simulink model "QFTAxiLite"  (R2023b)
settings: Solver=VariableStepAuto  StartTime=0.0  StopTime=30  FixedStep=0.01  RelTol=1e-3
undefined symbols (not defined in the file): AXI4, i, Lite
libraries: hdlBasic x224, vmcUtilities x1
(part 1 of 2)
settings Model: Creator=finla  LastModifiedBy=finla

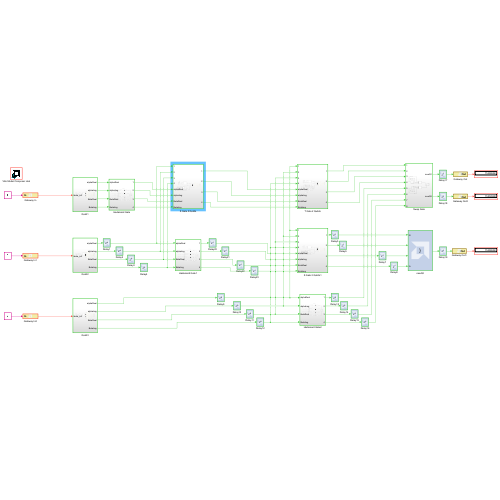
[thumbnail: Simulink's stored preview of the top-level diagram]
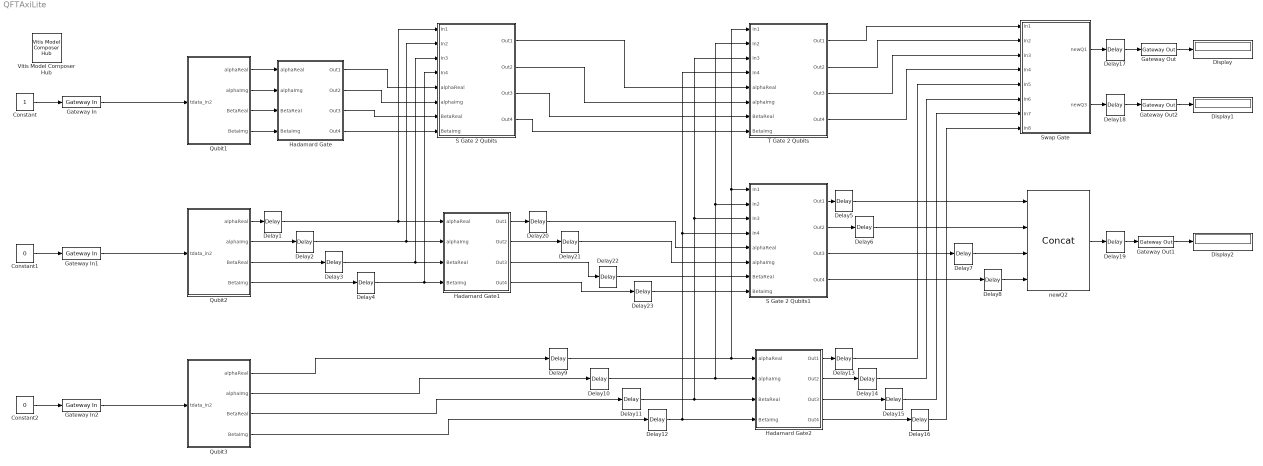
== system QFTAxiLite ==
  Constant : Constant
  Constant1 : Constant  Value=0
  Constant2 : Constant  Value=0
  Delay{1..4} (4 alike) : hdlBasic/Delay  rst=off  en=off  latency=4  reg_retiming=off  XmcBlockStatus=1  maskContainerNames=group1  block_type=delay  block_config=sysgen:Delay_config
  Delay{9..12} (4 alike) : hdlBasic/Delay  rst=off  en=off  latency=9  reg_retiming=off  XmcBlockStatus=1  maskContainerNames=group1  block_type=delay  block_config=sysgen:Delay_config
  Delay{13..16} (4 alike) : hdlBasic/Delay  rst=off  en=off  latency=2  reg_retiming=off  XmcBlockStatus=1  maskContainerNames=group1  block_type=delay  block_config=sysgen:Delay_config
  Delay{5..8,17..23} (11 alike) : hdlBasic/Delay  rst=off  en=off  latency=1  reg_retiming=off  XmcBlockStatus=1  maskContainerNames=group1  block_type=delay  block_config=sysgen:Delay_config
  Display : Display
  Display1 : Display
  Display2 : Display
  Gateway In : hdlBasic/Gateway In  gui_display_data_type=Fixed-point  arith_type=Unsigned  n_bits=32  bin_pt=0  preci_type=Single  exp_width=8  frac_width=24  rows=1  columns=1  quantization="Round  (unbiased: +/- Inf)"  overflow=Saturate  period=1  UseAsADC=off  ADCChannel='1'  interface=AXI4-Lite  automatic_assignment=on  address_offset=hex2dec('00')  intf_name=''  intf_description=''  default_value=0  timing_constraint=None  locs_specified=off  LOCs={}  io_standard={}  inherit_from_input=off  hdl_port=on  XmcBlockStatus=1  maskContainerNames=group4  block_type=gatewayin  block_config=sysgen:gateway_in_config  block_width_w=590  block_height_w=620  block_width=640  block_height=850
  Gateway In1 : hdlBasic/Gateway In  gui_display_data_type=Fixed-point  arith_type=Unsigned  n_bits=32  bin_pt=0  preci_type=Single  exp_width=8  frac_width=24  rows=1  columns=1  quantization="Round  (unbiased: +/- Inf)"  overflow=Saturate  period=1  UseAsADC=off  ADCChannel='1'  interface=AXI4-Lite  automatic_assignment=on  address_offset=hex2dec('00')  intf_name=''  intf_description=''  default_value=0  timing_constraint=None  locs_specified=off  LOCs={}  io_standard={}  inherit_from_input=off  hdl_port=on  XmcBlockStatus=1  maskContainerNames=group4  block_type=gatewayin  block_config=sysgen:gateway_in_config  block_width_w=590  block_height_w=620  block_width=640  block_height=850
  Gateway In2 : hdlBasic/Gateway In  gui_display_data_type=Fixed-point  arith_type=Unsigned  n_bits=32  bin_pt=0  preci_type=Single  exp_width=8  frac_width=24  rows=1  columns=1  quantization="Round  (unbiased: +/- Inf)"  overflow=Saturate  period=1  UseAsADC=off  ADCChannel='1'  interface=AXI4-Lite  automatic_assignment=on  address_offset=hex2dec('00')  intf_name=''  intf_description=''  default_value=0  timing_constraint=None  locs_specified=off  LOCs={}  io_standard={}  inherit_from_input=off  hdl_port=on  XmcBlockStatus=1  maskContainerNames=group4  block_type=gatewayin  block_config=sysgen:gateway_in_config  block_width_w=590  block_height_w=620  block_width=640  block_height=850
  Gateway Out : hdlBasic/Gateway Out  inherit_from_input=off  hdl_port=on  rows=1  columns=1  UseAsDAC=off  DACChannel='1'  interface=AXI4-Lite  automatic_assignment=on  address_offset=hex2dec('00')  intf_name=''  intf_description=''  timing_constraint=None  locs_specified=off  LOCs={}  io_standard={}  XmcBlockStatus=1  maskContainerNames=group4  block_type=gatewayout  block_config=sysgen:gateway_out_config  block_width_w=590  block_height_w=620  block_width=620  block_height=750
  Gateway Out1 : hdlBasic/Gateway Out  inherit_from_input=off  hdl_port=on  rows=1  columns=1  UseAsDAC=off  DACChannel='1'  interface=AXI4-Lite  automatic_assignment=on  address_offset=hex2dec('00')  intf_name=''  intf_description=''  timing_constraint=None  locs_specified=off  LOCs={}  io_standard={}  XmcBlockStatus=1  maskContainerNames=group4  block_type=gatewayout  block_config=sysgen:gateway_out_config  block_width_w=590  block_height_w=620  block_width=620  block_height=750
  Gateway Out2 : hdlBasic/Gateway Out  inherit_from_input=off  hdl_port=on  rows=1  columns=1  UseAsDAC=off  DACChannel='1'  interface=AXI4-Lite  automatic_assignment=on  address_offset=hex2dec('00')  intf_name=''  intf_description=''  timing_constraint=None  locs_specified=off  LOCs={}  io_standard={}  XmcBlockStatus=1  maskContainerNames=group4  block_type=gatewayout  block_config=sysgen:gateway_out_config  block_width_w=590  block_height_w=620  block_width=620  block_height=750
  Hadamard Gate : Subsystem
  Hadamard Gate1 : Subsystem
  Hadamard Gate2 : Subsystem
  Qubit1 : Subsystem
  Qubit2 : Subsystem
  Qubit3 : Subsystem
  S Gate 2 Qubits : Subsystem
  S Gate 2 Qubits1 : Subsystem
  Swap Gate : Subsystem
  T Gate 2 Qubits : Subsystem
  Vitis Model Composer Hub : vmcUtilities/Vitis Model Composer Hub  Tag=genX  CodeGeneration=off  SubsystemName=QFTAxiLite  CompilationType=HDLCompilation  ExportTypeV2=IP Catalog  TargetDirectory=C:/Users/finla/Documents/QuantumProject/GatesMCFiles/ThreeQubitQFT  exportDesign=off  analyzeDesign=on  validateDesignOnHw=off  ExportType=System Generator  IpVendor=xilinx.com  IpLibrary=hls  IpVersion=1.0  IpHWLanguage=Verilog  AieCompilerOptions={}  AieSimulatorOptions={}  CreateTestbench=off  TestbenchStackSize=10  RunRtlSim=off  RunCSim=off  RunAieSim=off  AieSimTimeout=50000  RunAieSimProfiling=off  LaunchVitisAnalyzer=off  PlotOutput=off  RunX86Sim=off  X86SimTimeout=10  GenHwImage=off  GenLibadfXo=off  GenHwValidationCode=off  PlatformType=Not Specified  HwSystemType=Baremetal  HwValidationTarget=hw  ProjDevice=xczu3eg-sbva484-1-i  ProjDevicePart=xczu3eg-sbva484-1-i  SamplePeriod=-1  ClockFrequency=200  DataPathParallelism=1  xilinxfamily=zynquplus  part=xczu3eg  speed=-1-i  package=sbva484  directory=C:/Users/finla/Documents/QuantumProject/GatesMCFiles/ThreeQubitQFT  testbench=on  incr_netlist=off  synthesis_tool=Vivado  clock_wrapper=Clock Enables  dbl_ovrd=According to Block Masks  dcm_input_clock_period=10  sysclk_period=10  simulink_period=1  eval_field=0  IPInfoJsonString="{\"HDLSubsystem\":{\"SubsystemName\":\"QFTAxiLite\",\"IPName\":\"axi_stream_template\",\"IPLibrary\":\"SysGen\",\"IPVendor\":\"strath.ac.uk\",\"IPVersion\":\"1.0\",\"TargetDirectory\":\"C:/Users/finla/Documents/QuantumProject/GatesMCFiles/ThreeQubitQFT\",\"SubsystemDir\":\"C:/Users/finla/Documents/QuantumProject/GatesMCFiles/ThreeQubitQFT\\\\ip\\\\QFTAxiLite\"},\"SubsystemTag\":\"HDLNode\"}"  LogFileName=''  NThreads=4
  newQ2 : hdlBasic/Concat  num_inputs=4  XmcBlockStatus=1  maskContainerNames=group1  block_type=concat  block_config=sysgen:Concat_config
  wires:
  Qubit2/1(alphaReal) -> Delay1/1
  Qubit3/3(BetaReal) -> Delay11/1
  Delay3/1 -> Hadamard Gate1/3(BetaReal), S Gate 2 Qubits/3(In3)
  Delay2/1 -> Hadamard Gate1/2(alphaImg), S Gate 2 Qubits/2(In2)
  T Gate 2 Qubits/3(Out3) -> Swap Gate/3(In3)
  Delay1/1 -> Hadamard Gate1/1(alphaReal), S Gate 2 Qubits/1(In1)
  Delay4/1 -> Hadamard Gate1/4(BetaImg), S Gate 2 Qubits/4(In4)
  newQ2/1 -> Delay19/1
  T Gate 2 Qubits/4(Out4) -> Swap Gate/4(In4)
  Hadamard Gate/1(Out1) -> S Gate 2 Qubits/5(alphaReal)
  Qubit1/1(alphaReal) -> Hadamard Gate/1(alphaReal)
  Qubit1/2(alphaImg) -> Hadamard Gate/2(alphaImg)
  Qubit3/4(BetaImg) -> Delay12/1
  S Gate 2 Qubits/1(Out1) -> T Gate 2 Qubits/5(alphaReal)
  Qubit1/3(BetaReal) -> Hadamard Gate/3(BetaReal)
  S Gate 2 Qubits/4(Out4) -> T Gate 2 Qubits/8(BetaImg)
  Swap Gate/2(newQ3) -> Delay18/1
  Qubit2/3(BetaReal) -> Delay3/1
  Gateway In1/1 -> Qubit2/1(tdata_in2)
  Hadamard Gate1/1(Out1) -> Delay20/1
  Qubit3/1(alphaReal) -> Delay9/1
  Hadamard Gate2/1(Out1) -> Delay13/1
  Gateway In/1 -> Qubit1/1(tdata_in2)
  Hadamard Gate2/3(Out3) -> Delay15/1
  Hadamard Gate2/2(Out2) -> Delay14/1
  Qubit1/4(BetaImg) -> Hadamard Gate/4(BetaImg)
  Delay10/1 -> Hadamard Gate2/2(alphaImg), S Gate 2 Qubits1/2(In2), T Gate 2 Qubits/2(In2)
  Hadamard Gate2/4(Out4) -> Delay16/1
  Qubit2/2(alphaImg) -> Delay2/1
  Hadamard Gate/3(Out3) -> S Gate 2 Qubits/7(BetaReal)
  Hadamard Gate/2(Out2) -> S Gate 2 Qubits/6(alphaImg)
  S Gate 2 Qubits/3(Out3) -> T Gate 2 Qubits/7(BetaReal)
  Delay11/1 -> Hadamard Gate2/3(BetaReal), S Gate 2 Qubits1/3(In3), T Gate 2 Qubits/3(In3)
  S Gate 2 Qubits/2(Out2) -> T Gate 2 Qubits/6(alphaImg)
  Delay12/1 -> Hadamard Gate2/4(BetaImg), S Gate 2 Qubits1/4(In4), T Gate 2 Qubits/4(In4)
  Hadamard Gate/4(Out4) -> S Gate 2 Qubits/8(BetaImg)
  Gateway In2/1 -> Qubit3/1(tdata_in2)
  Delay9/1 -> Hadamard Gate2/1(alphaReal), S Gate 2 Qubits1/1(In1), T Gate 2 Qubits/1(In1)
  Hadamard Gate1/2(Out2) -> Delay21/1
  Hadamard Gate1/4(Out4) -> Delay23/1
  Qubit3/2(alphaImg) -> Delay10/1
  Qubit2/4(BetaImg) -> Delay4/1
  Hadamard Gate1/3(Out3) -> Delay22/1
  Constant/1 -> Gateway In/1
  Constant1/1 -> Gateway In1/1
  Constant2/1 -> Gateway In2/1
  Gateway Out/1 -> Display/1
  Gateway Out2/1 -> Display1/1
  Gateway Out1/1 -> Display2/1
  Delay17/1 -> Gateway Out/1
  Delay18/1 -> Gateway Out2/1
  Delay19/1 -> Gateway Out1/1
  S Gate 2 Qubits1/1(Out1) -> Delay5/1
  S Gate 2 Qubits1/2(Out2) -> Delay6/1
  S Gate 2 Qubits1/3(Out3) -> Delay7/1
  S Gate 2 Qubits1/4(Out4) -> Delay8/1
  T Gate 2 Qubits/1(Out1) -> Swap Gate/1(In1)
  T Gate 2 Qubits/2(Out2) -> Swap Gate/2(In2)
  Delay13/1 -> Swap Gate/5(In5)
  Delay14/1 -> Swap Gate/6(In6)
  Delay15/1 -> Swap Gate/7(In7)
  Delay16/1 -> Swap Gate/8(In8)
  Swap Gate/1(newQ1) -> Delay17/1
  Delay20/1 -> S Gate 2 Qubits1/5(alphaReal)
  Delay21/1 -> S Gate 2 Qubits1/6(alphaImg)
  Delay22/1 -> S Gate 2 Qubits1/7(BetaReal)
  Delay23/1 -> S Gate 2 Qubits1/8(BetaImg)
  Delay5/1 -> newQ2/1
  Delay6/1 -> newQ2/2
  Delay7/1 -> newQ2/3
  Delay8/1 -> newQ2/4

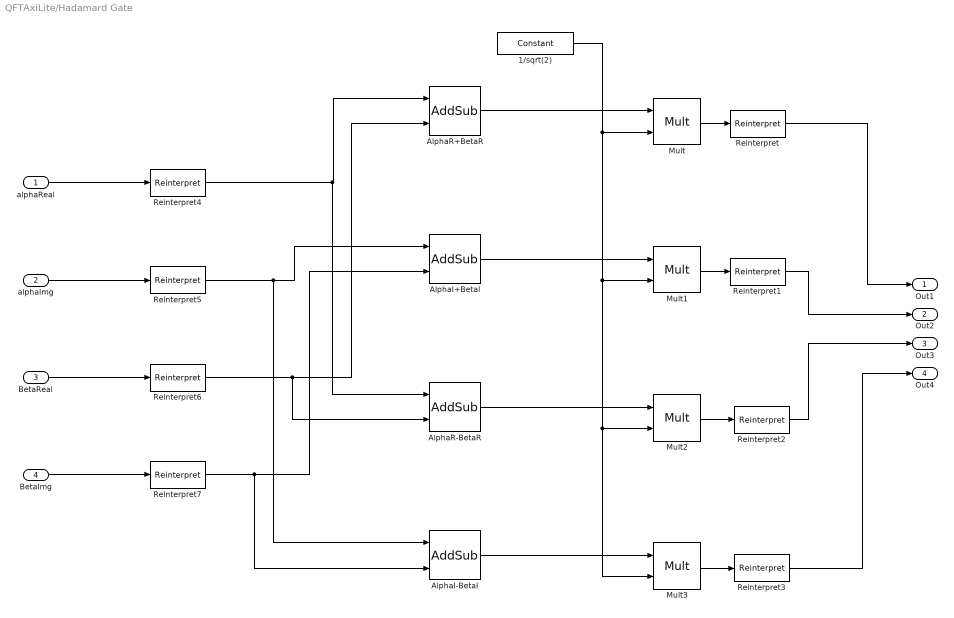
== system QFTAxiLite/Hadamard Gate ==
  alphaReal : Inport
  alphaImg : Inport  Port=2
  BetaReal : Inport  Port=3
  BetaImg : Inport  Port=4
  1/sqrt(2) : hdlBasic/Constant  const=1/sqrt(2)  gui_display_data_type=Fixed-point  arith_type=Signed (2's comp)  n_bits=16  bin_pt=13  preci_type=Single  exp_width=8  frac_width=24  explicit_period=on  period=1  XmcBlockStatus=1  maskContainerNames=tabcontainer1  block_type=constant  block_config=sysgen:Constant_config
  AlphaI+BetaI : hdlBasic/AddSub  mode=Addition  use_carryin=off  use_carryout=off  en=off  latency=1  precision=User Defined  arith_type="Signed  (2's comp)"  n_bits=8  bin_pt=0  quantization=Truncate  overflow=Saturate  use_behavioral_HDL=off  hw_selection=Fabric  pipelined=off  XmcBlockStatus=1  maskContainerNames=tabcontainer1  block_type=addsub  block_config=sysgen:Addsub_config
  AlphaI-BetaI : hdlBasic/AddSub  mode=Subtraction  use_carryin=off  use_carryout=off  en=off  latency=1  precision=User Defined  arith_type="Signed  (2's comp)"  n_bits=8  bin_pt=0  quantization=Truncate  overflow=Saturate  use_behavioral_HDL=off  hw_selection=Fabric  pipelined=off  XmcBlockStatus=1  maskContainerNames=tabcontainer1  block_type=addsub  block_config=sysgen:Addsub_config
  AlphaR+BetaR : hdlBasic/AddSub  mode=Addition  use_carryin=off  use_carryout=off  en=off  latency=1  precision=User Defined  arith_type="Signed  (2's comp)"  n_bits=8  bin_pt=0  quantization=Truncate  overflow=Saturate  use_behavioral_HDL=off  hw_selection=Fabric  pipelined=off  XmcBlockStatus=1  maskContainerNames=tabcontainer1  block_type=addsub  block_config=sysgen:Addsub_config
  AlphaR-BetaR : hdlBasic/AddSub  mode=Subtraction  use_carryin=off  use_carryout=off  en=off  latency=1  precision=User Defined  arith_type="Signed  (2's comp)"  n_bits=8  bin_pt=0  quantization=Truncate  overflow=Saturate  use_behavioral_HDL=off  hw_selection=Fabric  pipelined=off  XmcBlockStatus=1  maskContainerNames=tabcontainer1  block_type=addsub  block_config=sysgen:Addsub_config
  Mult{,1..3} (4 alike) : hdlBasic/Mult  precision=User Defined  arith_type="Signed  (2's comp)"  n_bits=8  bin_pt=6  quantization=Truncate  overflow=Flag as error  en=off  latency=3  use_behavioral_HDL=off  opt=Speed  use_embedded=on  optimum_pipeline=off  pipeline=on  use_rpm=on  placement_style=Triangular  XmcBlockStatus=1  maskContainerNames=group1  block_type=mult  block_config=sysgen:Mult_config  block_width=598  block_height=876
  Reinterpret{,1..3} (4 alike) : hdlBasic/Reinterpret  force_arith_type=on  arith_type=Unsigned  force_bin_pt=on  bin_pt=0  XmcBlockStatus=1  maskContainerNames=group1  block_type=reinterpret  block_config=sysgen:Reinterpret_config
  Reinterpret{4..7} (4 alike) : hdlBasic/Reinterpret  force_arith_type=on  arith_type="Signed  (2's comp)"  force_bin_pt=off  bin_pt=0  XmcBlockStatus=1  maskContainerNames=group1  block_type=reinterpret  block_config=sysgen:Reinterpret_config
  Out1 : Outport
  Out2 : Outport  Port=2
  Out3 : Outport  Port=3
  Out4 : Outport  Port=4
  wires:
  Reinterpret/1 -> Out1/1
  AlphaI-BetaI/1 -> Mult3/1
  Mult1/1 -> Reinterpret1/1
  Mult/1 -> Reinterpret/1
  Mult3/1 -> Reinterpret3/1
  Reinterpret3/1 -> Out4/1
  Reinterpret1/1 -> Out2/1
  AlphaR-BetaR/1 -> Mult2/1
  1/sqrt(2)/1 -> Mult3/2, Mult2/2, Mult1/2, Mult/2
  Reinterpret2/1 -> Out3/1
  AlphaI+BetaI/1 -> Mult1/1
  Mult2/1 -> Reinterpret2/1
  AlphaR+BetaR/1 -> Mult/1
  alphaReal/1 -> Reinterpret4/1
  alphaImg/1 -> Reinterpret5/1
  BetaReal/1 -> Reinterpret6/1
  BetaImg/1 -> Reinterpret7/1
  Reinterpret4/1 -> AlphaR-BetaR/1, AlphaR+BetaR/1
  Reinterpret5/1 -> AlphaI-BetaI/1, AlphaI+BetaI/1
  Reinterpret6/1 -> AlphaR-BetaR/2, AlphaR+BetaR/2
  Reinterpret7/1 -> AlphaI-BetaI/2, AlphaI+BetaI/2

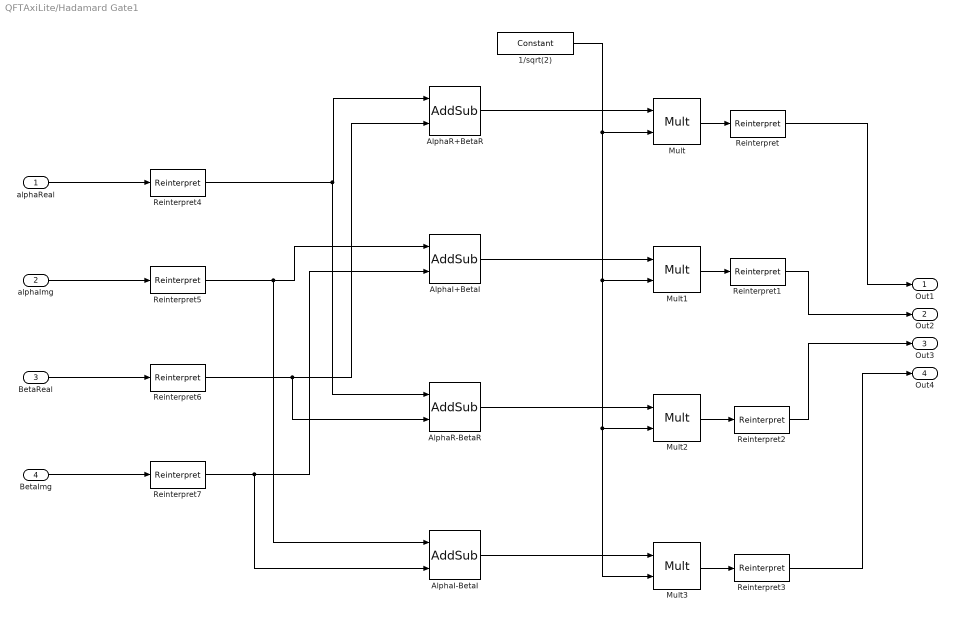
== system QFTAxiLite/Hadamard Gate1 ==
  alphaReal : Inport
  alphaImg : Inport  Port=2
  BetaReal : Inport  Port=3
  BetaImg : Inport  Port=4
  1/sqrt(2) : hdlBasic/Constant  const=1/sqrt(2)  gui_display_data_type=Fixed-point  arith_type=Signed (2's comp)  n_bits=16  bin_pt=13  preci_type=Single  exp_width=8  frac_width=24  explicit_period=on  period=1  XmcBlockStatus=1  maskContainerNames=tabcontainer1  block_type=constant  block_config=sysgen:Constant_config
  AlphaI+BetaI : hdlBasic/AddSub  mode=Addition  use_carryin=off  use_carryout=off  en=off  latency=1  precision=User Defined  arith_type="Signed  (2's comp)"  n_bits=8  bin_pt=0  quantization=Truncate  overflow=Saturate  use_behavioral_HDL=off  hw_selection=Fabric  pipelined=off  XmcBlockStatus=1  maskContainerNames=tabcontainer1  block_type=addsub  block_config=sysgen:Addsub_config
  AlphaI-BetaI : hdlBasic/AddSub  mode=Subtraction  use_carryin=off  use_carryout=off  en=off  latency=1  precision=User Defined  arith_type="Signed  (2's comp)"  n_bits=8  bin_pt=0  quantization=Truncate  overflow=Saturate  use_behavioral_HDL=off  hw_selection=Fabric  pipelined=off  XmcBlockStatus=1  maskContainerNames=tabcontainer1  block_type=addsub  block_config=sysgen:Addsub_config
  AlphaR+BetaR : hdlBasic/AddSub  mode=Addition  use_carryin=off  use_carryout=off  en=off  latency=1  precision=User Defined  arith_type="Signed  (2's comp)"  n_bits=8  bin_pt=0  quantization=Truncate  overflow=Saturate  use_behavioral_HDL=off  hw_selection=Fabric  pipelined=off  XmcBlockStatus=1  maskContainerNames=tabcontainer1  block_type=addsub  block_config=sysgen:Addsub_config
  AlphaR-BetaR : hdlBasic/AddSub  mode=Subtraction  use_carryin=off  use_carryout=off  en=off  latency=1  precision=User Defined  arith_type="Signed  (2's comp)"  n_bits=8  bin_pt=0  quantization=Truncate  overflow=Saturate  use_behavioral_HDL=off  hw_selection=Fabric  pipelined=off  XmcBlockStatus=1  maskContainerNames=tabcontainer1  block_type=addsub  block_config=sysgen:Addsub_config
  Mult{,1..3} (4 alike) : hdlBasic/Mult  precision=User Defined  arith_type="Signed  (2's comp)"  n_bits=8  bin_pt=6  quantization=Truncate  overflow=Flag as error  en=off  latency=3  use_behavioral_HDL=off  opt=Speed  use_embedded=on  optimum_pipeline=off  pipeline=on  use_rpm=on  placement_style=Triangular  XmcBlockStatus=1  maskContainerNames=group1  block_type=mult  block_config=sysgen:Mult_config  block_width=598  block_height=876
  Reinterpret{,1..3} (4 alike) : hdlBasic/Reinterpret  force_arith_type=on  arith_type=Unsigned  force_bin_pt=on  bin_pt=0  XmcBlockStatus=1  maskContainerNames=group1  block_type=reinterpret  block_config=sysgen:Reinterpret_config
  Reinterpret{4..7} (4 alike) : hdlBasic/Reinterpret  force_arith_type=on  arith_type="Signed  (2's comp)"  force_bin_pt=off  bin_pt=0  XmcBlockStatus=1  maskContainerNames=group1  block_type=reinterpret  block_config=sysgen:Reinterpret_config
  Out1 : Outport
  Out2 : Outport  Port=2
  Out3 : Outport  Port=3
  Out4 : Outport  Port=4
  wires:
  Reinterpret/1 -> Out1/1
  AlphaI-BetaI/1 -> Mult3/1
  Mult1/1 -> Reinterpret1/1
  Mult/1 -> Reinterpret/1
  Mult3/1 -> Reinterpret3/1
  Reinterpret3/1 -> Out4/1
  Reinterpret1/1 -> Out2/1
  AlphaR-BetaR/1 -> Mult2/1
  1/sqrt(2)/1 -> Mult3/2, Mult2/2, Mult1/2, Mult/2
  Reinterpret2/1 -> Out3/1
  AlphaI+BetaI/1 -> Mult1/1
  Mult2/1 -> Reinterpret2/1
  AlphaR+BetaR/1 -> Mult/1
  alphaReal/1 -> Reinterpret4/1
  alphaImg/1 -> Reinterpret5/1
  BetaReal/1 -> Reinterpret6/1
  BetaImg/1 -> Reinterpret7/1
  Reinterpret4/1 -> AlphaR-BetaR/1, AlphaR+BetaR/1
  Reinterpret5/1 -> AlphaI-BetaI/1, AlphaI+BetaI/1
  Reinterpret6/1 -> AlphaR-BetaR/2, AlphaR+BetaR/2
  Reinterpret7/1 -> AlphaI-BetaI/2, AlphaI+BetaI/2

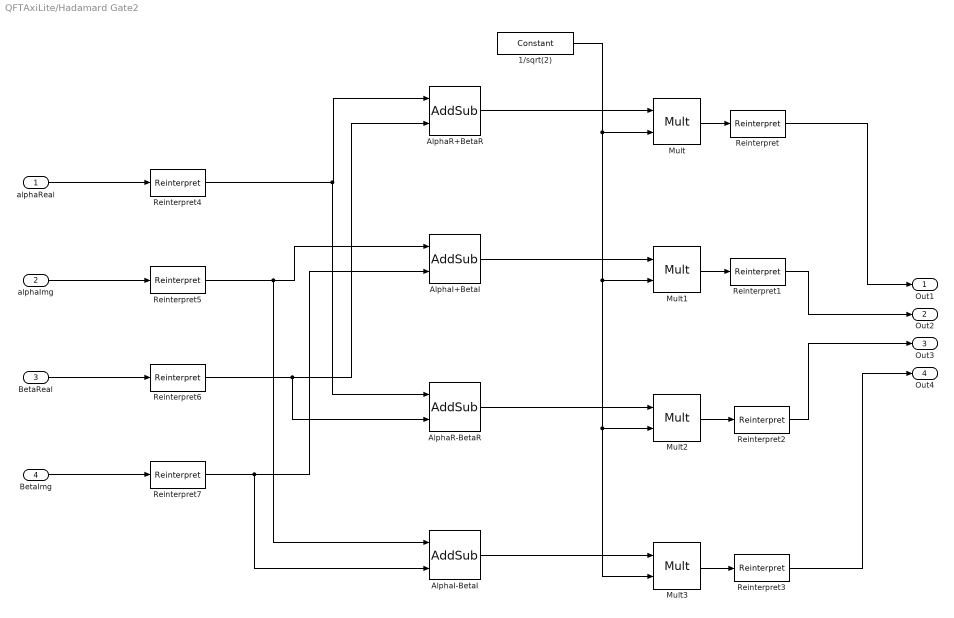
== system QFTAxiLite/Hadamard Gate2 ==
  alphaReal : Inport
  alphaImg : Inport  Port=2
  BetaReal : Inport  Port=3
  BetaImg : Inport  Port=4
  1/sqrt(2) : hdlBasic/Constant  const=1/sqrt(2)  gui_display_data_type=Fixed-point  arith_type=Signed (2's comp)  n_bits=16  bin_pt=13  preci_type=Single  exp_width=8  frac_width=24  explicit_period=on  period=1  XmcBlockStatus=1  maskContainerNames=tabcontainer1  block_type=constant  block_config=sysgen:Constant_config
  AlphaI+BetaI : hdlBasic/AddSub  mode=Addition  use_carryin=off  use_carryout=off  en=off  latency=1  precision=User Defined  arith_type="Signed  (2's comp)"  n_bits=8  bin_pt=0  quantization=Truncate  overflow=Saturate  use_behavioral_HDL=off  hw_selection=Fabric  pipelined=off  XmcBlockStatus=1  maskContainerNames=tabcontainer1  block_type=addsub  block_config=sysgen:Addsub_config
  AlphaI-BetaI : hdlBasic/AddSub  mode=Subtraction  use_carryin=off  use_carryout=off  en=off  latency=1  precision=User Defined  arith_type="Signed  (2's comp)"  n_bits=8  bin_pt=0  quantization=Truncate  overflow=Saturate  use_behavioral_HDL=off  hw_selection=Fabric  pipelined=off  XmcBlockStatus=1  maskContainerNames=tabcontainer1  block_type=addsub  block_config=sysgen:Addsub_config
  AlphaR+BetaR : hdlBasic/AddSub  mode=Addition  use_carryin=off  use_carryout=off  en=off  latency=1  precision=User Defined  arith_type="Signed  (2's comp)"  n_bits=8  bin_pt=0  quantization=Truncate  overflow=Saturate  use_behavioral_HDL=off  hw_selection=Fabric  pipelined=off  XmcBlockStatus=1  maskContainerNames=tabcontainer1  block_type=addsub  block_config=sysgen:Addsub_config
  AlphaR-BetaR : hdlBasic/AddSub  mode=Subtraction  use_carryin=off  use_carryout=off  en=off  latency=1  precision=User Defined  arith_type="Signed  (2's comp)"  n_bits=8  bin_pt=0  quantization=Truncate  overflow=Saturate  use_behavioral_HDL=off  hw_selection=Fabric  pipelined=off  XmcBlockStatus=1  maskContainerNames=tabcontainer1  block_type=addsub  block_config=sysgen:Addsub_config
  Mult{,1..3} (4 alike) : hdlBasic/Mult  precision=User Defined  arith_type="Signed  (2's comp)"  n_bits=8  bin_pt=6  quantization=Truncate  overflow=Flag as error  en=off  latency=3  use_behavioral_HDL=off  opt=Speed  use_embedded=on  optimum_pipeline=off  pipeline=on  use_rpm=on  placement_style=Triangular  XmcBlockStatus=1  maskContainerNames=group1  block_type=mult  block_config=sysgen:Mult_config  block_width=598  block_height=876
  Reinterpret{,1..3} (4 alike) : hdlBasic/Reinterpret  force_arith_type=on  arith_type=Unsigned  force_bin_pt=on  bin_pt=0  XmcBlockStatus=1  maskContainerNames=group1  block_type=reinterpret  block_config=sysgen:Reinterpret_config
  Reinterpret{4..7} (4 alike) : hdlBasic/Reinterpret  force_arith_type=on  arith_type="Signed  (2's comp)"  force_bin_pt=off  bin_pt=0  XmcBlockStatus=1  maskContainerNames=group1  block_type=reinterpret  block_config=sysgen:Reinterpret_config
  Out1 : Outport
  Out2 : Outport  Port=2
  Out3 : Outport  Port=3
  Out4 : Outport  Port=4
  wires:
  Reinterpret/1 -> Out1/1
  AlphaI-BetaI/1 -> Mult3/1
  Mult1/1 -> Reinterpret1/1
  Mult/1 -> Reinterpret/1
  Mult3/1 -> Reinterpret3/1
  Reinterpret3/1 -> Out4/1
  Reinterpret1/1 -> Out2/1
  AlphaR-BetaR/1 -> Mult2/1
  1/sqrt(2)/1 -> Mult3/2, Mult2/2, Mult1/2, Mult/2
  Reinterpret2/1 -> Out3/1
  AlphaI+BetaI/1 -> Mult1/1
  Mult2/1 -> Reinterpret2/1
  AlphaR+BetaR/1 -> Mult/1
  alphaReal/1 -> Reinterpret4/1
  alphaImg/1 -> Reinterpret5/1
  BetaReal/1 -> Reinterpret6/1
  BetaImg/1 -> Reinterpret7/1
  Reinterpret4/1 -> AlphaR-BetaR/1, AlphaR+BetaR/1
  Reinterpret5/1 -> AlphaI-BetaI/1, AlphaI+BetaI/1
  Reinterpret6/1 -> AlphaR-BetaR/2, AlphaR+BetaR/2
  Reinterpret7/1 -> AlphaI-BetaI/2, AlphaI+BetaI/2

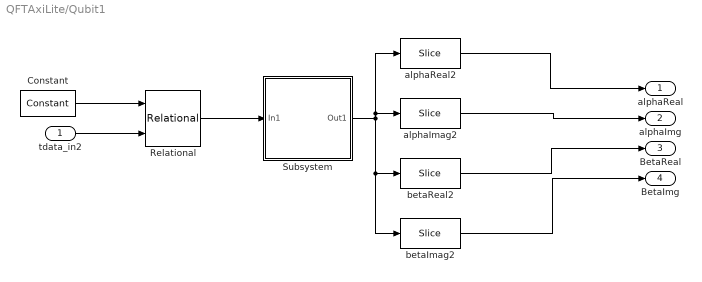
== system QFTAxiLite/Qubit1 ==
  tdata_in2 : Inport
  Constant : hdlBasic/Constant  const=0.0  gui_display_data_type=Fixed-point  arith_type=Unsigned  n_bits=32  bin_pt=0  preci_type=Single  exp_width=8  frac_width=24  explicit_period=off  period=1  XmcBlockStatus=1  maskContainerNames=tabcontainer1  block_type=constant  block_config=sysgen:Constant_config
  Relational : hdlBasic/Relational  mode=a=b  op_type=Unsigned Fix  en=off  latency=1  XmcBlockStatus=1  maskContainerNames=tabcontainer1  block_type=relational  block_config=sysgen:Relational_config
  Subsystem : Subsystem
  alphaImag2 : hdlBasic/Slice  nbits=16  boolean_output=off  mode=Two Bit Locations  bit1=23  base1=LSB of Input  bit0=16  base0=LSB of Input  XmcBlockStatus=1  maskContainerNames=group1  block_type=slice  block_config=sysgen:Slice_config
  alphaReal2 : hdlBasic/Slice  nbits=16  boolean_output=off  mode=Two Bit Locations  bit1=31  base1=LSB of Input  bit0=24  base0=LSB of Input  XmcBlockStatus=1  maskContainerNames=group1  block_type=slice  block_config=sysgen:Slice_config
  betaImag2 : hdlBasic/Slice  nbits=16  boolean_output=off  mode=Two Bit Locations  bit1=7  base1=LSB of Input  bit0=0  base0=LSB of Input  XmcBlockStatus=1  maskContainerNames=group1  block_type=slice  block_config=sysgen:Slice_config
  betaReal2 : hdlBasic/Slice  nbits=16  boolean_output=off  mode=Two Bit Locations  bit1=15  base1=LSB of Input  bit0=8  base0=LSB of Input  XmcBlockStatus=1  maskContainerNames=group1  block_type=slice  block_config=sysgen:Slice_config
  alphaReal : Outport
  alphaImg : Outport  Port=2
  BetaReal : Outport  Port=3
  BetaImg : Outport  Port=4
  wires:
  tdata_in2/1 -> Relational/2
  Constant/1 -> Relational/1
  Relational/1 -> Subsystem/1(In1)
  betaImag2/1 -> BetaImg/1
  betaReal2/1 -> BetaReal/1
  alphaReal2/1 -> alphaReal/1
  alphaImag2/1 -> alphaImg/1
  Subsystem/1(Out1) -> betaImag2/1, betaReal2/1, alphaImag2/1, alphaReal2/1

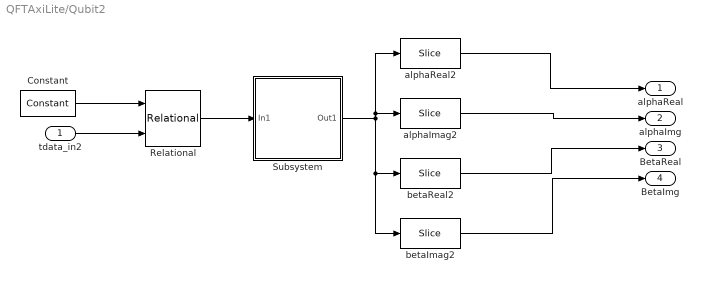
== system QFTAxiLite/Qubit2 ==
  tdata_in2 : Inport
  Constant : hdlBasic/Constant  const=0.0  gui_display_data_type=Fixed-point  arith_type=Unsigned  n_bits=32  bin_pt=0  preci_type=Single  exp_width=8  frac_width=24  explicit_period=off  period=1  XmcBlockStatus=1  maskContainerNames=tabcontainer1  block_type=constant  block_config=sysgen:Constant_config
  Relational : hdlBasic/Relational  mode=a=b  op_type=Unsigned Fix  en=off  latency=1  XmcBlockStatus=1  maskContainerNames=tabcontainer1  block_type=relational  block_config=sysgen:Relational_config
  Subsystem : Subsystem
  alphaImag2 : hdlBasic/Slice  nbits=16  boolean_output=off  mode=Two Bit Locations  bit1=23  base1=LSB of Input  bit0=16  base0=LSB of Input  XmcBlockStatus=1  maskContainerNames=group1  block_type=slice  block_config=sysgen:Slice_config
  alphaReal2 : hdlBasic/Slice  nbits=16  boolean_output=off  mode=Two Bit Locations  bit1=31  base1=LSB of Input  bit0=24  base0=LSB of Input  XmcBlockStatus=1  maskContainerNames=group1  block_type=slice  block_config=sysgen:Slice_config
  betaImag2 : hdlBasic/Slice  nbits=16  boolean_output=off  mode=Two Bit Locations  bit1=7  base1=LSB of Input  bit0=0  base0=LSB of Input  XmcBlockStatus=1  maskContainerNames=group1  block_type=slice  block_config=sysgen:Slice_config
  betaReal2 : hdlBasic/Slice  nbits=16  boolean_output=off  mode=Two Bit Locations  bit1=15  base1=LSB of Input  bit0=8  base0=LSB of Input  XmcBlockStatus=1  maskContainerNames=group1  block_type=slice  block_config=sysgen:Slice_config
  alphaReal : Outport
  alphaImg : Outport  Port=2
  BetaReal : Outport  Port=3
  BetaImg : Outport  Port=4
  wires:
  tdata_in2/1 -> Relational/2
  Constant/1 -> Relational/1
  Relational/1 -> Subsystem/1(In1)
  betaImag2/1 -> BetaImg/1
  betaReal2/1 -> BetaReal/1
  alphaReal2/1 -> alphaReal/1
  alphaImag2/1 -> alphaImg/1
  Subsystem/1(Out1) -> betaImag2/1, betaReal2/1, alphaImag2/1, alphaReal2/1

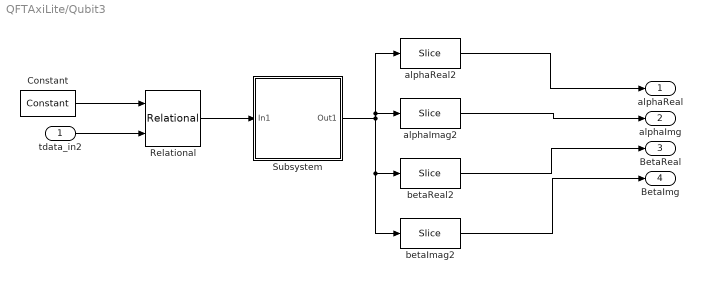
== system QFTAxiLite/Qubit3 ==
  tdata_in2 : Inport
  Constant : hdlBasic/Constant  const=0.0  gui_display_data_type=Fixed-point  arith_type=Unsigned  n_bits=32  bin_pt=0  preci_type=Single  exp_width=8  frac_width=24  explicit_period=off  period=1  XmcBlockStatus=1  maskContainerNames=tabcontainer1  block_type=constant  block_config=sysgen:Constant_config
  Relational : hdlBasic/Relational  mode=a=b  op_type=Unsigned Fix  en=off  latency=1  XmcBlockStatus=1  maskContainerNames=tabcontainer1  block_type=relational  block_config=sysgen:Relational_config
  Subsystem : Subsystem
  alphaImag2 : hdlBasic/Slice  nbits=16  boolean_output=off  mode=Two Bit Locations  bit1=23  base1=LSB of Input  bit0=16  base0=LSB of Input  XmcBlockStatus=1  maskContainerNames=group1  block_type=slice  block_config=sysgen:Slice_config
  alphaReal2 : hdlBasic/Slice  nbits=16  boolean_output=off  mode=Two Bit Locations  bit1=31  base1=LSB of Input  bit0=24  base0=LSB of Input  XmcBlockStatus=1  maskContainerNames=group1  block_type=slice  block_config=sysgen:Slice_config
  betaImag2 : hdlBasic/Slice  nbits=16  boolean_output=off  mode=Two Bit Locations  bit1=7  base1=LSB of Input  bit0=0  base0=LSB of Input  XmcBlockStatus=1  maskContainerNames=group1  block_type=slice  block_config=sysgen:Slice_config
  betaReal2 : hdlBasic/Slice  nbits=16  boolean_output=off  mode=Two Bit Locations  bit1=15  base1=LSB of Input  bit0=8  base0=LSB of Input  XmcBlockStatus=1  maskContainerNames=group1  block_type=slice  block_config=sysgen:Slice_config
  alphaReal : Outport
  alphaImg : Outport  Port=2
  BetaReal : Outport  Port=3
  BetaImg : Outport  Port=4
  wires:
  tdata_in2/1 -> Relational/2
  Constant/1 -> Relational/1
  Relational/1 -> Subsystem/1(In1)
  betaImag2/1 -> BetaImg/1
  betaReal2/1 -> BetaReal/1
  alphaReal2/1 -> alphaReal/1
  alphaImag2/1 -> alphaImg/1
  Subsystem/1(Out1) -> betaImag2/1, betaReal2/1, alphaImag2/1, alphaReal2/1

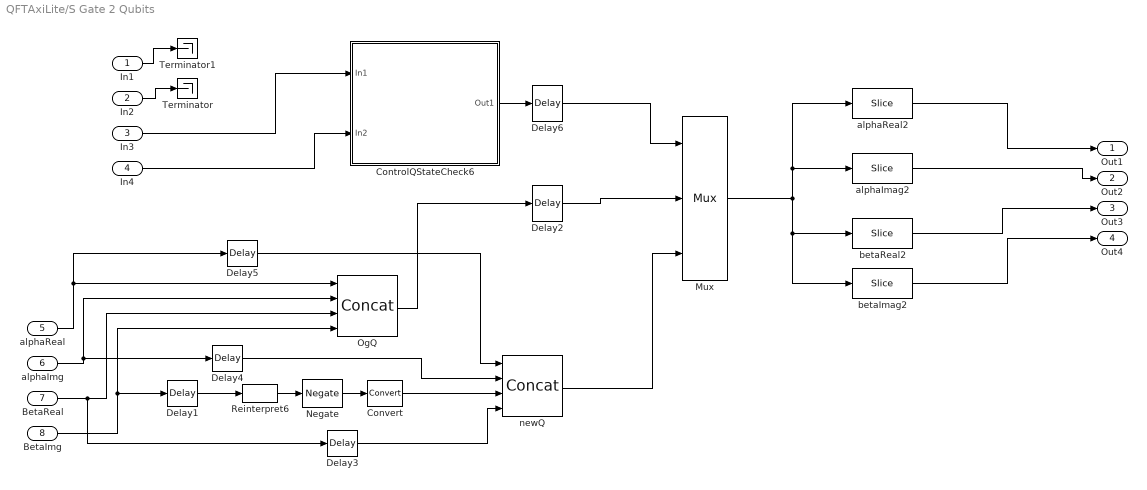
== system QFTAxiLite/S Gate 2 Qubits ==
  In1 : Inport
  In2 : Inport  Port=2
  In3 : Inport  Port=3
  In4 : Inport  Port=4
  alphaReal : Inport  Port=5
  alphaImg : Inport  Port=6
  BetaReal : Inport  Port=7
  BetaImg : Inport  Port=8
  ControlQStateCheck6 : Subsystem
  Convert : hdlBasic/Convert  gui_display_data_type=Fixed-point  arith_type=Unsigned  n_bits=8  bin_pt=0  float_type=Single  exp_bits=8  fraction_bits=24  quantization=Truncate  overflow=Wrap  en=off  latency=1  pipeline=off  XmcBlockStatus=1  maskContainerNames=group2  block_type=convert  block_config=sysgen:Convert_config  block_width=595  block_height=885
  Delay1 : hdlBasic/Delay  rst=off  en=off  latency=2  reg_retiming=off  XmcBlockStatus=1  maskContainerNames=group1  block_type=delay  block_config=sysgen:Delay_config
  Delay{2..5} (4 alike) : hdlBasic/Delay  rst=off  en=off  latency=4  reg_retiming=off  XmcBlockStatus=1  maskContainerNames=group1  block_type=delay  block_config=sysgen:Delay_config
  Delay6 : hdlBasic/Delay  rst=off  en=off  latency=1  reg_retiming=off  XmcBlockStatus=1  maskContainerNames=group1  block_type=delay  block_config=sysgen:Delay_config
  Mux : hdlBasic/Mux  inputs=2  en=off  latency=1  precision=Full  arith_type=Unsigned  n_bits=16  bin_pt=14  quantization=Truncate  overflow=Wrap  XmcBlockStatus=1  maskContainerNames=tabcontainer1  block_type=mux  block_config=sysgen:Mux_config
  Negate : hdlBasic/Negate  precision=Full  arith_type=Unsigned  n_bits=16  bin_pt=14  quantization=Truncate  overflow=Wrap  en=off  latency=1  XmcBlockStatus=1  maskContainerNames=tabcontainer1  block_type=negate  block_config=sysgen:Negate_config
  OgQ : hdlBasic/Concat  num_inputs=4  XmcBlockStatus=1  maskContainerNames=group1  block_type=concat  block_config=sysgen:Concat_config
  Reinterpret6 : hdlBasic/Reinterpret  force_arith_type=on  arith_type="Signed  (2's comp)"  force_bin_pt=off  bin_pt=0  XmcBlockStatus=1  maskContainerNames=group1  block_type=reinterpret  block_config=sysgen:Reinterpret_config
  Terminator : Terminator
  Terminator1 : Terminator
  alphaImag2 : hdlBasic/Slice  nbits=16  boolean_output=off  mode=Two Bit Locations  bit1=23  base1=LSB of Input  bit0=16  base0=LSB of Input  XmcBlockStatus=1  maskContainerNames=group1  block_type=slice  block_config=sysgen:Slice_config
  alphaReal2 : hdlBasic/Slice  nbits=16  boolean_output=off  mode=Two Bit Locations  bit1=31  base1=LSB of Input  bit0=24  base0=LSB of Input  XmcBlockStatus=1  maskContainerNames=group1  block_type=slice  block_config=sysgen:Slice_config
  betaImag2 : hdlBasic/Slice  nbits=16  boolean_output=off  mode=Two Bit Locations  bit1=7  base1=LSB of Input  bit0=0  base0=LSB of Input  XmcBlockStatus=1  maskContainerNames=group1  block_type=slice  block_config=sysgen:Slice_config
  betaReal2 : hdlBasic/Slice  nbits=16  boolean_output=off  mode=Two Bit Locations  bit1=15  base1=LSB of Input  bit0=8  base0=LSB of Input  XmcBlockStatus=1  maskContainerNames=group1  block_type=slice  block_config=sysgen:Slice_config
  newQ : hdlBasic/Concat  num_inputs=4  XmcBlockStatus=1  maskContainerNames=group1  block_type=concat  block_config=sysgen:Concat_config
  Out1 : Outport
  Out2 : Outport  Port=2
  Out3 : Outport  Port=3
  Out4 : Outport  Port=4
  wires:
  In3/1 -> ControlQStateCheck6/1(In1)
  In4/1 -> ControlQStateCheck6/2(In2)
  OgQ/1 -> Delay2/1
  ControlQStateCheck6/1(Out1) -> Delay6/1
  In1/1 -> Terminator1/1
  Delay2/1 -> Mux/2
  Delay3/1 -> newQ/4
  Convert/1 -> newQ/3
  alphaImag2/1 -> Out2/1
  betaImag2/1 -> Out4/1
  Mux/1 -> betaImag2/1, betaReal2/1, alphaImag2/1, alphaReal2/1
  alphaReal2/1 -> Out1/1
  betaReal2/1 -> Out3/1
  alphaReal/1 -> OgQ/1, Delay5/1
  alphaImg/1 -> OgQ/2, Delay4/1
  BetaReal/1 -> OgQ/3, Delay3/1
  BetaImg/1 -> OgQ/4, Delay1/1
  In2/1 -> Terminator/1
  Reinterpret6/1 -> Negate/1
  Delay1/1 -> Reinterpret6/1
  Delay4/1 -> newQ/2
  newQ/1 -> Mux/3
  Delay6/1 -> Mux/1
  Delay5/1 -> newQ/1
  Negate/1 -> Convert/1

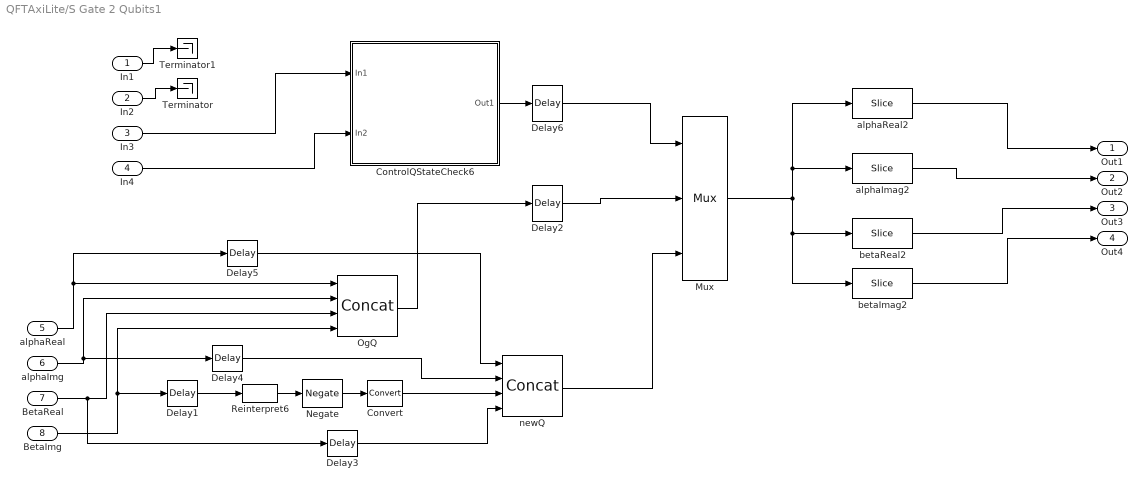
== system QFTAxiLite/S Gate 2 Qubits1 ==
  In1 : Inport
  In2 : Inport  Port=2
  In3 : Inport  Port=3
  In4 : Inport  Port=4
  alphaReal : Inport  Port=5
  alphaImg : Inport  Port=6
  BetaReal : Inport  Port=7
  BetaImg : Inport  Port=8
  ControlQStateCheck6 : Subsystem
  Convert : hdlBasic/Convert  gui_display_data_type=Fixed-point  arith_type=Unsigned  n_bits=8  bin_pt=0  float_type=Single  exp_bits=8  fraction_bits=24  quantization=Truncate  overflow=Wrap  en=off  latency=1  pipeline=off  XmcBlockStatus=1  maskContainerNames=group2  block_type=convert  block_config=sysgen:Convert_config  block_width=595  block_height=885
  Delay1 : hdlBasic/Delay  rst=off  en=off  latency=2  reg_retiming=off  XmcBlockStatus=1  maskContainerNames=group1  block_type=delay  block_config=sysgen:Delay_config
  Delay{2..5} (4 alike) : hdlBasic/Delay  rst=off  en=off  latency=4  reg_retiming=off  XmcBlockStatus=1  maskContainerNames=group1  block_type=delay  block_config=sysgen:Delay_config
  Delay6 : hdlBasic/Delay  rst=off  en=off  latency=1  reg_retiming=off  XmcBlockStatus=1  maskContainerNames=group1  block_type=delay  block_config=sysgen:Delay_config
  Mux : hdlBasic/Mux  inputs=2  en=off  latency=1  precision=Full  arith_type=Unsigned  n_bits=16  bin_pt=14  quantization=Truncate  overflow=Wrap  XmcBlockStatus=1  maskContainerNames=tabcontainer1  block_type=mux  block_config=sysgen:Mux_config
  Negate : hdlBasic/Negate  precision=Full  arith_type=Unsigned  n_bits=16  bin_pt=14  quantization=Truncate  overflow=Wrap  en=off  latency=1  XmcBlockStatus=1  maskContainerNames=tabcontainer1  block_type=negate  block_config=sysgen:Negate_config
  OgQ : hdlBasic/Concat  num_inputs=4  XmcBlockStatus=1  maskContainerNames=group1  block_type=concat  block_config=sysgen:Concat_config
  Reinterpret6 : hdlBasic/Reinterpret  force_arith_type=on  arith_type="Signed  (2's comp)"  force_bin_pt=off  bin_pt=0  XmcBlockStatus=1  maskContainerNames=group1  block_type=reinterpret  block_config=sysgen:Reinterpret_config
  Terminator : Terminator
  Terminator1 : Terminator
  alphaImag2 : hdlBasic/Slice  nbits=16  boolean_output=off  mode=Two Bit Locations  bit1=23  base1=LSB of Input  bit0=16  base0=LSB of Input  XmcBlockStatus=1  maskContainerNames=group1  block_type=slice  block_config=sysgen:Slice_config
  alphaReal2 : hdlBasic/Slice  nbits=16  boolean_output=off  mode=Two Bit Locations  bit1=31  base1=LSB of Input  bit0=24  base0=LSB of Input  XmcBlockStatus=1  maskContainerNames=group1  block_type=slice  block_config=sysgen:Slice_config
  betaImag2 : hdlBasic/Slice  nbits=16  boolean_output=off  mode=Two Bit Locations  bit1=7  base1=LSB of Input  bit0=0  base0=LSB of Input  XmcBlockStatus=1  maskContainerNames=group1  block_type=slice  block_config=sysgen:Slice_config
  betaReal2 : hdlBasic/Slice  nbits=16  boolean_output=off  mode=Two Bit Locations  bit1=15  base1=LSB of Input  bit0=8  base0=LSB of Input  XmcBlockStatus=1  maskContainerNames=group1  block_type=slice  block_config=sysgen:Slice_config
  newQ : hdlBasic/Concat  num_inputs=4  XmcBlockStatus=1  maskContainerNames=group1  block_type=concat  block_config=sysgen:Concat_config
  Out1 : Outport
  Out2 : Outport  Port=2
  Out3 : Outport  Port=3
  Out4 : Outport  Port=4
  wires:
  In3/1 -> ControlQStateCheck6/1(In1)
  In4/1 -> ControlQStateCheck6/2(In2)
  OgQ/1 -> Delay2/1
  ControlQStateCheck6/1(Out1) -> Delay6/1
  In1/1 -> Terminator1/1
  Delay2/1 -> Mux/2
  Delay3/1 -> newQ/4
  Convert/1 -> newQ/3
  alphaImag2/1 -> Out2/1
  betaImag2/1 -> Out4/1
  Mux/1 -> betaImag2/1, betaReal2/1, alphaImag2/1, alphaReal2/1
  alphaReal2/1 -> Out1/1
  betaReal2/1 -> Out3/1
  alphaReal/1 -> OgQ/1, Delay5/1
  alphaImg/1 -> OgQ/2, Delay4/1
  BetaReal/1 -> OgQ/3, Delay3/1
  BetaImg/1 -> OgQ/4, Delay1/1
  In2/1 -> Terminator/1
  Reinterpret6/1 -> Negate/1
  Delay1/1 -> Reinterpret6/1
  Delay4/1 -> newQ/2
  newQ/1 -> Mux/3
  Delay6/1 -> Mux/1
  Delay5/1 -> newQ/1
  Negate/1 -> Convert/1

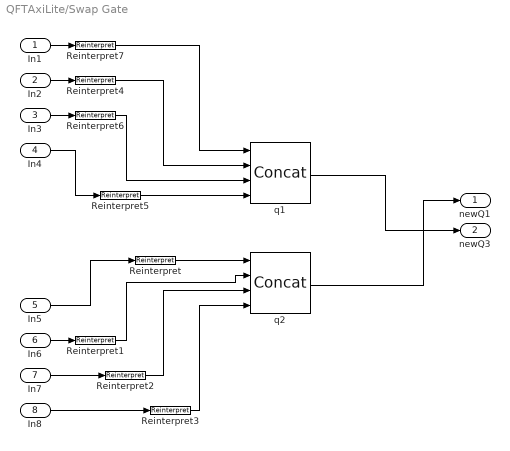
== system QFTAxiLite/Swap Gate ==
  In1 : Inport
  In2 : Inport  Port=2
  In3 : Inport  Port=3
  In4 : Inport  Port=4
  In5 : Inport  Port=5
  In6 : Inport  Port=6
  In7 : Inport  Port=7
  In8 : Inport  Port=8
  Reinterpret{,1..7} (8 alike) : hdlBasic/Reinterpret  force_arith_type=on  arith_type=Unsigned  force_bin_pt=off  bin_pt=0  XmcBlockStatus=1  maskContainerNames=group1  block_type=reinterpret  block_config=sysgen:Reinterpret_config
  q1 : hdlBasic/Concat  num_inputs=4  XmcBlockStatus=1  maskContainerNames=group1  block_type=concat  block_config=sysgen:Concat_config
  q2 : hdlBasic/Concat  num_inputs=4  XmcBlockStatus=1  maskContainerNames=group1  block_type=concat  block_config=sysgen:Concat_config
  newQ1 : Outport
  newQ3 : Outport  Port=2
  wires:
  In7/1 -> Reinterpret2/1
  q1/1 -> newQ3/1
  In6/1 -> Reinterpret1/1
  q2/1 -> newQ1/1
  In4/1 -> Reinterpret5/1
  In3/1 -> Reinterpret6/1
  In8/1 -> Reinterpret3/1
  In5/1 -> Reinterpret/1
  In2/1 -> Reinterpret4/1
  In1/1 -> Reinterpret7/1
  Reinterpret/1 -> q2/1
  Reinterpret3/1 -> q2/4
  Reinterpret1/1 -> q2/2
  Reinterpret2/1 -> q2/3
  Reinterpret5/1 -> q1/4
  Reinterpret6/1 -> q1/3
  Reinterpret4/1 -> q1/2
  Reinterpret7/1 -> q1/1

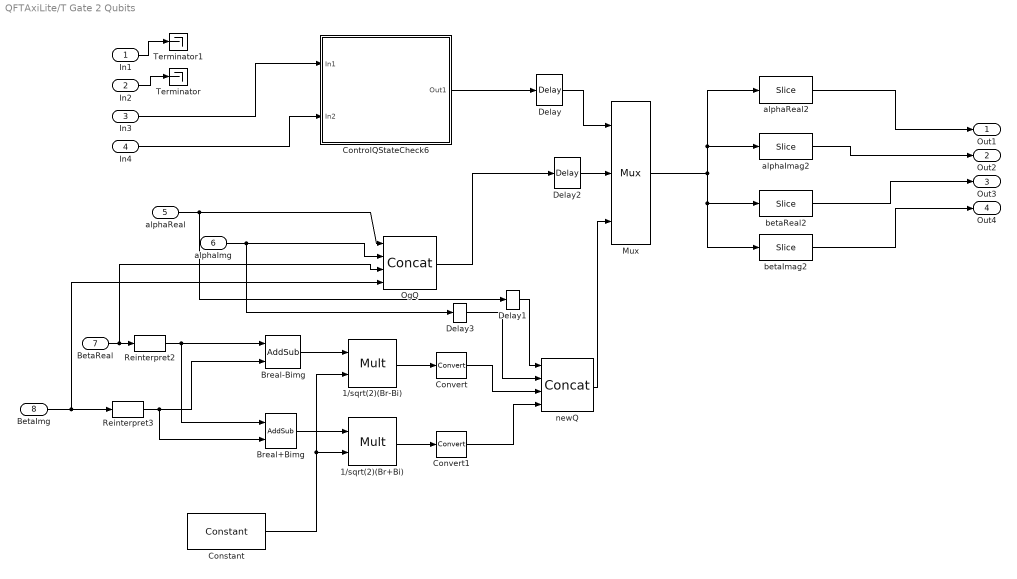
== system QFTAxiLite/T Gate 2 Qubits ==
  In1 : Inport
  In2 : Inport  Port=2
  In3 : Inport  Port=3
  In4 : Inport  Port=4
  alphaReal : Inport  Port=5
  alphaImg : Inport  Port=6
  BetaReal : Inport  Port=7
  BetaImg : Inport  Port=8
  1/sqrt(2)(Br+Bi) : hdlBasic/Mult  precision=Full  arith_type="Signed  (2's comp)"  n_bits=8  bin_pt=6  quantization=Truncate  overflow=Wrap  en=off  latency=3  use_behavioral_HDL=off  opt=Speed  use_embedded=on  optimum_pipeline=off  pipeline=on  use_rpm=on  placement_style=Triangular  XmcBlockStatus=1  maskContainerNames=group1  block_type=mult  block_config=sysgen:Mult_config  block_width=598  block_height=876
  1/sqrt(2)(Br-Bi) : hdlBasic/Mult  precision=Full  arith_type="Signed  (2's comp)"  n_bits=8  bin_pt=6  quantization=Truncate  overflow=Wrap  en=off  latency=3  use_behavioral_HDL=off  opt=Speed  use_embedded=on  optimum_pipeline=off  pipeline=on  use_rpm=on  placement_style=Triangular  XmcBlockStatus=1  maskContainerNames=group1  block_type=mult  block_config=sysgen:Mult_config  block_width=598  block_height=876
  Breal+Bimg : hdlBasic/AddSub  mode=Addition  use_carryin=off  use_carryout=off  en=off  latency=1  precision=Full  arith_type=Unsigned  n_bits=8  bin_pt=6  quantization=Truncate  overflow=Wrap  use_behavioral_HDL=off  hw_selection=Fabric  pipelined=off  XmcBlockStatus=1  maskContainerNames=tabcontainer1  block_type=addsub  block_config=sysgen:Addsub_config
  Breal-Bimg : hdlBasic/AddSub  mode=Subtraction  use_carryin=off  use_carryout=off  en=off  latency=1  precision=Full  arith_type=Unsigned  n_bits=8  bin_pt=6  quantization=Truncate  overflow=Wrap  use_behavioral_HDL=off  hw_selection=Fabric  pipelined=off  XmcBlockStatus=1  maskContainerNames=tabcontainer1  block_type=addsub  block_config=sysgen:Addsub_config
  Constant : hdlBasic/Constant  const=1/sqrt(2)  gui_display_data_type=Fixed-point  arith_type=Signed (2's comp)  n_bits=16  bin_pt=13  preci_type=Single  exp_width=8  frac_width=24  explicit_period=off  period=1  XmcBlockStatus=1  maskContainerNames=tabcontainer1  block_type=constant  block_config=sysgen:Constant_config
  ControlQStateCheck6 : Subsystem
  Convert : hdlBasic/Convert  gui_display_data_type=Fixed-point  arith_type=Unsigned  n_bits=8  bin_pt=0  float_type=Single  exp_bits=8  fraction_bits=24  quantization=Truncate  overflow=Wrap  en=off  latency=1  pipeline=off  XmcBlockStatus=1  maskContainerNames=group2  block_type=convert  block_config=sysgen:Convert_config  block_width=595  block_height=885
  Convert1 : hdlBasic/Convert  gui_display_data_type=Fixed-point  arith_type=Unsigned  n_bits=8  bin_pt=0  float_type=Single  exp_bits=8  fraction_bits=24  quantization=Truncate  overflow=Wrap  en=off  latency=1  pipeline=off  XmcBlockStatus=1  maskContainerNames=group2  block_type=convert  block_config=sysgen:Convert_config  block_width=595  block_height=885
  Delay : hdlBasic/Delay  rst=off  en=off  latency=2  reg_retiming=off  XmcBlockStatus=1  maskContainerNames=group1  block_type=delay  block_config=sysgen:Delay_config
  Delay1 : hdlBasic/Delay  rst=off  en=off  latency=5  reg_retiming=off  XmcBlockStatus=1  maskContainerNames=group1  block_type=delay  block_config=sysgen:Delay_config
  Delay2 : hdlBasic/Delay  rst=off  en=off  latency=5  reg_retiming=off  XmcBlockStatus=1  maskContainerNames=group1  block_type=delay  block_config=sysgen:Delay_config
  Delay3 : hdlBasic/Delay  rst=off  en=off  latency=5  reg_retiming=off  XmcBlockStatus=1  maskContainerNames=group1  block_type=delay  block_config=sysgen:Delay_config
  Mux : hdlBasic/Mux  inputs=2  en=off  latency=1  precision=Full  arith_type=Unsigned  n_bits=16  bin_pt=14  quantization=Truncate  overflow=Wrap  XmcBlockStatus=1  maskContainerNames=tabcontainer1  block_type=mux  block_config=sysgen:Mux_config
  OgQ : hdlBasic/Concat  num_inputs=4  XmcBlockStatus=1  maskContainerNames=group1  block_type=concat  block_config=sysgen:Concat_config
  Reinterpret2 : hdlBasic/Reinterpret  force_arith_type=on  arith_type="Signed  (2's comp)"  force_bin_pt=off  bin_pt=0  XmcBlockStatus=1  maskContainerNames=group1  block_type=reinterpret  block_config=sysgen:Reinterpret_config
  Reinterpret3 : hdlBasic/Reinterpret  force_arith_type=on  arith_type="Signed  (2's comp)"  force_bin_pt=off  bin_pt=0  XmcBlockStatus=1  maskContainerNames=group1  block_type=reinterpret  block_config=sysgen:Reinterpret_config
  Terminator : Terminator
  Terminator1 : Terminator
  alphaImag2 : hdlBasic/Slice  nbits=16  boolean_output=off  mode=Two Bit Locations  bit1=23  base1=LSB of Input  bit0=16  base0=LSB of Input  XmcBlockStatus=1  maskContainerNames=group1  block_type=slice  block_config=sysgen:Slice_config
  alphaReal2 : hdlBasic/Slice  nbits=16  boolean_output=off  mode=Two Bit Locations  bit1=31  base1=LSB of Input  bit0=24  base0=LSB of Input  XmcBlockStatus=1  maskContainerNames=group1  block_type=slice  block_config=sysgen:Slice_config
  betaImag2 : hdlBasic/Slice  nbits=16  boolean_output=off  mode=Two Bit Locations  bit1=7  base1=LSB of Input  bit0=0  base0=LSB of Input  XmcBlockStatus=1  maskContainerNames=group1  block_type=slice  block_config=sysgen:Slice_config
  betaReal2 : hdlBasic/Slice  nbits=16  boolean_output=off  mode=Two Bit Locations  bit1=15  base1=LSB of Input  bit0=8  base0=LSB of Input  XmcBlockStatus=1  maskContainerNames=group1  block_type=slice  block_config=sysgen:Slice_config
  newQ : hdlBasic/Concat  num_inputs=4  XmcBlockStatus=1  maskContainerNames=group1  block_type=concat  block_config=sysgen:Concat_config
  Out1 : Outport
  Out2 : Outport  Port=2
  Out3 : Outport  Port=3
  Out4 : Outport  Port=4
  wires:
  ControlQStateCheck6/1(Out1) -> Delay/1
  In3/1 -> ControlQStateCheck6/1(In1)
  In4/1 -> ControlQStateCheck6/2(In2)
  In2/1 -> Terminator/1
  Mux/1 -> betaImag2/1, betaReal2/1, alphaImag2/1, alphaReal2/1
  BetaImg/1 -> OgQ/4, Reinterpret3/1
  alphaReal/1 -> Delay1/1, OgQ/1
  newQ/1 -> Mux/3
  1/sqrt(2)(Br-Bi)/1 -> Convert/1
  BetaReal/1 -> OgQ/3, Reinterpret2/1
  alphaReal2/1 -> Out1/1
  OgQ/1 -> Delay2/1
  In1/1 -> Terminator1/1
  alphaImag2/1 -> Out2/1
  1/sqrt(2)(Br+Bi)/1 -> Convert1/1
  betaImag2/1 -> Out4/1
  alphaImg/1 -> Delay3/1, OgQ/2
  betaReal2/1 -> Out3/1
  Delay2/1 -> Mux/2
  Constant/1 -> 1/sqrt(2)(Br-Bi)/2, 1/sqrt(2)(Br+Bi)/2
  Breal+Bimg/1 -> 1/sqrt(2)(Br+Bi)/1
  Breal-Bimg/1 -> 1/sqrt(2)(Br-Bi)/1
  Delay/1 -> Mux/1
  Delay1/1 -> newQ/1
  Delay3/1 -> newQ/2
  Reinterpret2/1 -> Breal+Bimg/1, Breal-Bimg/1
  Reinterpret3/1 -> Breal-Bimg/2, Breal+Bimg/2
  Convert/1 -> newQ/3
  Convert1/1 -> newQ/4

== system QFTAxiLite/Qubit1/Subsystem ==
  In1 : Inport
  Delay5 : hdlBasic/Delay  rst=off  en=off  latency=1  reg_retiming=off  XmcBlockStatus=1  maskContainerNames=group1  block_type=delay  block_config=sysgen:Delay_config
  Is0 : Subsystem
  Is1 : Subsystem
  Mux : hdlBasic/Mux  inputs=2  en=off  latency=1  precision=Full  arith_type=Unsigned  n_bits=16  bin_pt=14  quantization=Truncate  overflow=Wrap  XmcBlockStatus=1  maskContainerNames=tabcontainer1  block_type=mux  block_config=sysgen:Mux_config
  Out1 : Outport
  wires:
  Mux/1 -> Out1/1
  In1/1 -> Delay5/1
  Delay5/1 -> Mux/1
  Is1/1(Out1) -> Mux/2
  Is0/1(Out1) -> Mux/3

== system QFTAxiLite/Qubit2/Subsystem ==
  In1 : Inport
  Delay1 : hdlBasic/Delay  rst=off  en=off  latency=1  reg_retiming=off  XmcBlockStatus=1  maskContainerNames=group1  block_type=delay  block_config=sysgen:Delay_config
  Delay2 : hdlBasic/Delay  rst=off  en=off  latency=1  reg_retiming=off  XmcBlockStatus=1  maskContainerNames=group1  block_type=delay  block_config=sysgen:Delay_config
  Delay5 : hdlBasic/Delay  rst=off  en=off  latency=1  reg_retiming=off  XmcBlockStatus=1  maskContainerNames=group1  block_type=delay  block_config=sysgen:Delay_config
  Is0 : Subsystem
  Is1 : Subsystem
  Mux : hdlBasic/Mux  inputs=2  en=off  latency=1  precision=Full  arith_type=Unsigned  n_bits=16  bin_pt=14  quantization=Truncate  overflow=Wrap  XmcBlockStatus=1  maskContainerNames=tabcontainer1  block_type=mux  block_config=sysgen:Mux_config
  Out1 : Outport
  wires:
  Is1/1(Out1) -> Delay1/1
  Mux/1 -> Out1/1
  Is0/1(Out1) -> Delay2/1
  In1/1 -> Delay5/1
  Delay5/1 -> Mux/1
  Delay1/1 -> Mux/2
  Delay2/1 -> Mux/3

== system QFTAxiLite/Qubit3/Subsystem ==
  In1 : Inport
  Delay1 : hdlBasic/Delay  rst=off  en=off  latency=1  reg_retiming=off  XmcBlockStatus=1  maskContainerNames=group1  block_type=delay  block_config=sysgen:Delay_config
  Delay2 : hdlBasic/Delay  rst=off  en=off  latency=1  reg_retiming=off  XmcBlockStatus=1  maskContainerNames=group1  block_type=delay  block_config=sysgen:Delay_config
  Delay5 : hdlBasic/Delay  rst=off  en=off  latency=1  reg_retiming=off  XmcBlockStatus=1  maskContainerNames=group1  block_type=delay  block_config=sysgen:Delay_config
  Is0 : Subsystem
  Is1 : Subsystem
  Mux : hdlBasic/Mux  inputs=2  en=off  latency=1  precision=Full  arith_type=Unsigned  n_bits=16  bin_pt=14  quantization=Truncate  overflow=Wrap  XmcBlockStatus=1  maskContainerNames=tabcontainer1  block_type=mux  block_config=sysgen:Mux_config
  Out1 : Outport
  wires:
  Is1/1(Out1) -> Delay1/1
  Mux/1 -> Out1/1
  Is0/1(Out1) -> Delay2/1
  In1/1 -> Delay5/1
  Delay5/1 -> Mux/1
  Delay1/1 -> Mux/2
  Delay2/1 -> Mux/3

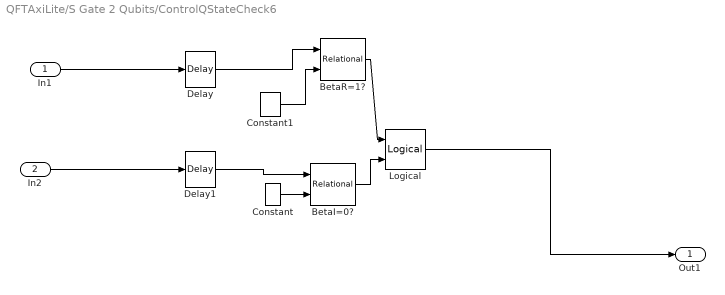
== system QFTAxiLite/S Gate 2 Qubits/ControlQStateCheck6 ==
  In1 : Inport
  In2 : Inport  Port=2
  BetaI=0? : hdlBasic/Relational  mode=a=b  op_type=Unsigned Fix  en=off  latency=1  XmcBlockStatus=1  maskContainerNames=tabcontainer1  block_type=relational  block_config=sysgen:Relational_config
  BetaR=1? : hdlBasic/Relational  mode=a=b  op_type=Unsigned Fix  en=off  latency=1  XmcBlockStatus=1  maskContainerNames=tabcontainer1  block_type=relational  block_config=sysgen:Relational_config
  Constant : hdlBasic/Constant  const=0  gui_display_data_type=Fixed-point  arith_type=Unsigned  n_bits=8  bin_pt=6  preci_type=Single  exp_width=8  frac_width=24  explicit_period=off  period=1  XmcBlockStatus=1  maskContainerNames=tabcontainer1  block_type=constant  block_config=sysgen:Constant_config
  Constant1 : hdlBasic/Constant  const=1  gui_display_data_type=Fixed-point  arith_type=Unsigned  n_bits=8  bin_pt=6  preci_type=Single  exp_width=8  frac_width=24  explicit_period=off  period=1  XmcBlockStatus=1  maskContainerNames=tabcontainer1  block_type=constant  block_config=sysgen:Constant_config
  Delay : hdlBasic/Delay  rst=off  en=off  latency=1  reg_retiming=off  XmcBlockStatus=1  maskContainerNames=group1  block_type=delay  block_config=sysgen:Delay_config
  Delay1 : hdlBasic/Delay  rst=off  en=off  latency=1  reg_retiming=off  XmcBlockStatus=1  maskContainerNames=group1  block_type=delay  block_config=sysgen:Delay_config
  Logical : hdlBasic/Logical  logical_function=AND  inputs=2  en=off  latency=1  precision=Full  arith_type=Unsigned  n_bits=16  bin_pt=0  align_bp=on  overflow=[]  quantization=[]  XmcBlockStatus=1  maskContainerNames=tabcontainer1  block_type=logical  block_config=sysgen:Logical_config
  Out1 : Outport
  wires:
  BetaI=0?/1 -> Logical/2
  In1/1 -> Delay/1
  Constant/1 -> BetaI=0?/2
  Delay1/1 -> BetaI=0?/1
  Logical/1 -> Out1/1
  Constant1/1 -> BetaR=1?/2
  BetaR=1?/1 -> Logical/1
  Delay/1 -> BetaR=1?/1
  In2/1 -> Delay1/1

== system QFTAxiLite/S Gate 2 Qubits1/ControlQStateCheck6 ==
  In1 : Inport
  In2 : Inport  Port=2
  BetaI=0? : hdlBasic/Relational  mode=a=b  op_type=Unsigned Fix  en=off  latency=1  XmcBlockStatus=1  maskContainerNames=tabcontainer1  block_type=relational  block_config=sysgen:Relational_config
  BetaR=1? : hdlBasic/Relational  mode=a=b  op_type=Unsigned Fix  en=off  latency=1  XmcBlockStatus=1  maskContainerNames=tabcontainer1  block_type=relational  block_config=sysgen:Relational_config
  Constant : hdlBasic/Constant  const=0  gui_display_data_type=Fixed-point  arith_type=Unsigned  n_bits=8  bin_pt=6  preci_type=Single  exp_width=8  frac_width=24  explicit_period=off  period=1  XmcBlockStatus=1  maskContainerNames=tabcontainer1  block_type=constant  block_config=sysgen:Constant_config
  Constant1 : hdlBasic/Constant  const=1  gui_display_data_type=Fixed-point  arith_type=Unsigned  n_bits=8  bin_pt=6  preci_type=Single  exp_width=8  frac_width=24  explicit_period=off  period=1  XmcBlockStatus=1  maskContainerNames=tabcontainer1  block_type=constant  block_config=sysgen:Constant_config
  Delay : hdlBasic/Delay  rst=off  en=off  latency=1  reg_retiming=off  XmcBlockStatus=1  maskContainerNames=group1  block_type=delay  block_config=sysgen:Delay_config
  Delay1 : hdlBasic/Delay  rst=off  en=off  latency=1  reg_retiming=off  XmcBlockStatus=1  maskContainerNames=group1  block_type=delay  block_config=sysgen:Delay_config
  Logical : hdlBasic/Logical  logical_function=AND  inputs=2  en=off  latency=1  precision=Full  arith_type=Unsigned  n_bits=16  bin_pt=0  align_bp=on  overflow=[]  quantization=[]  XmcBlockStatus=1  maskContainerNames=tabcontainer1  block_type=logical  block_config=sysgen:Logical_config
  Out1 : Outport
  wires:
  BetaI=0?/1 -> Logical/2
  In1/1 -> Delay/1
  Constant/1 -> BetaI=0?/2
  Delay1/1 -> BetaI=0?/1
  Logical/1 -> Out1/1
  Constant1/1 -> BetaR=1?/2
  BetaR=1?/1 -> Logical/1
  Delay/1 -> BetaR=1?/1
  In2/1 -> Delay1/1
